simulink model "ExceptionGenerator"  (R2021b)
settings: Solver=FixedStepAuto  StartTime=0.0  StopTime=Inf  FixedStep=0.01  RelTol=1e-3
settings Model: Creator=MKlev  LastModifiedBy=MKlev
settings OptimizationCC: LocalBlockOutputs=off  ZeroExternalMemoryAtStartup=off  ZeroInternalMemoryAtStartup=off
settings RTWCC: Description=TwinCAT GRT Target  SystemTargetFile=TwinCatGrt.tlc  GenCodeOnly=on  TemplateMakefile=tcgrt_msbuild.tmf  TargetLang=C++
settings STFCustomTargetCC: TargetLangStandard=C++03 (ISO)  CombineOutputUpdateFcns=on  CodeInterfacePackaging=C++ class  CPPClassGenCompliant=on  GRTInterface=off  SystemTargetFile=TwinCatGrt.tlc
settings GRTTargetCC: TargetLangStandard=C++03 (ISO)  ParMdlRefBuildCompliant=off  CompOptLevelCompliant=off  ConcurrentExecutionCompliant=off  MatFileLogging=off  CodeInterfacePackaging=C++ class  UseToolchainInfoCompliant=off  ExtModeMexFile=TcExtModeClient

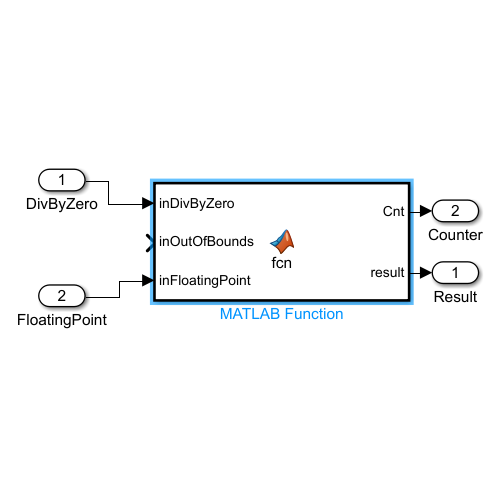
[thumbnail: Simulink's stored preview of the top-level diagram]
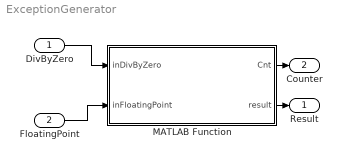
== system ExceptionGenerator ==
  DivByZero : Inport  OutDataTypeStr=boolean
  FloatingPoint : Inport  Port=2  OutDataTypeStr=boolean
  MATLAB Function : MATLAB Function  TreatAsAtomicUnit=on
  Result : Outport
  Counter : Outport  Port=2
  wires:
  DivByZero/1 -> MATLAB Function/1(inDivByZero)
  MATLAB Function/2(result) -> Result/1
  MATLAB Function/1(Cnt) -> Counter/1
  FloatingPoint/1 -> MATLAB Function/2(inFloatingPoint)

== matlab function ExceptionGenerator/MATLAB Function ==
  data: inDivByZero input; Cnt output; result output; inFloatingPoint input
function [Cnt,result]= fcn(inDivByZero, inFloatingPoint)

    persistent Counter a b fPosInf fNegInf
    if isempty(Counter)
        Counter = 0;
        a=1; 
        b=0;

        fNegInf = -1.7E+308 * 2;
        fPosInf = 1.7E+308 *2;
    end
    
    Counter = Counter+1; 
    
    if inDivByZero
       result = a/b; 
    elseif inFloatingPoint
        result = fPosInf + fNegInf;
    else
       result=0;
    end
    
Cnt=Counter;
